simulink model "Euler"  (R2023b)
settings: Solver=ode1  StartTime=0.0  StopTime=10.0  FixedStep=0.01  RelTol=1e-3
settings Model: Creator=Geo  LastModifiedBy=Geo

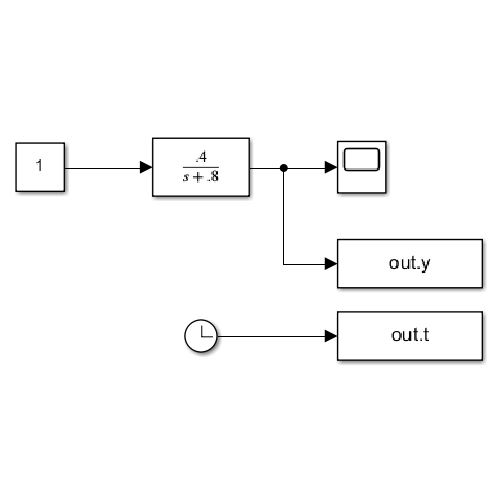
[thumbnail: Simulink's stored preview of the top-level diagram]
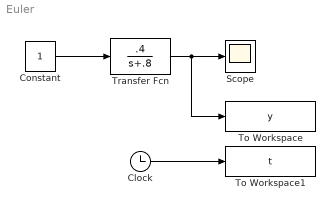
== system Euler ==
  Clock : Clock
  Constant : Constant
  Scope : Scope
  To Workspace : ToWorkspace  VariableName=y  SampleTime=-1
  To Workspace1 : ToWorkspace  VariableName=t  SampleTime=-1
  Transfer Fcn : TransferFcn  Numerator=[.4]  Denominator=[1 .8]
  wires:
  Constant/1 -> Transfer Fcn/1
  Transfer Fcn/1 -> To Workspace/1, Scope/1
  Clock/1 -> To Workspace1/1
